simulink model "21-E"  (R2014a)
settings: Solver=FixedStepDiscrete  StartTime=0.0  StopTime=10.0  FixedStep=0.0005  RelTol=1e-3
undefined symbols (not defined in the file): add_k1_100, add_k2_100, ADDspeed, cal_acc_div, cal_acc_flo_add, cal_acc_min, cal_an_div, cal_an_min, cal_bre_div, cal_bre_en_add, cal_bre_flo_add, cal_bre_min, cal_conf_off, cal_conf_on, controller, ecucoder_acal, enres_on_add, enres_per_add
libraries: simulink x165, ec55xxlib x29
(part 3 of 6)

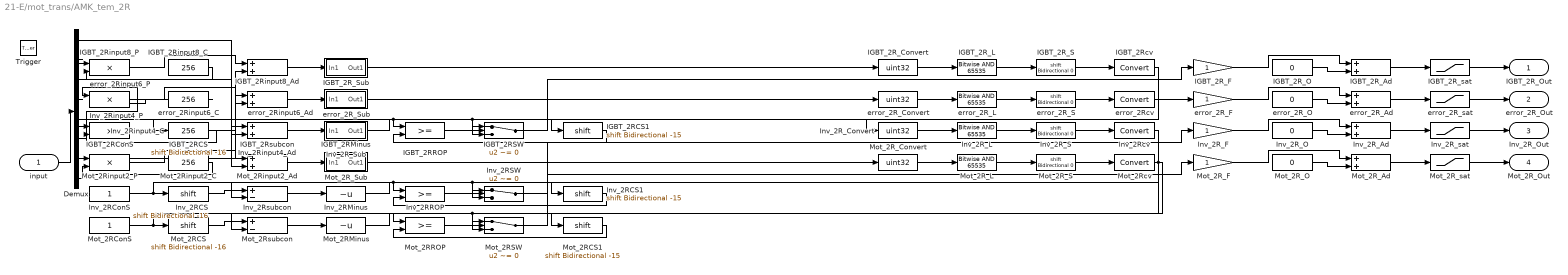
== system 21-E/mot_trans/AMK_tem_2R ==
  input : Inport
  Trigger : TriggerPort  TriggerType=function-call  PortDimensions=1
  Demux : Demux  Outputs=8
  IGBT_2RCS : ArithShift  BitShiftNumber=-16
  IGBT_2RCS1 : ArithShift  BitShiftNumber=-15
  IGBT_2RConS : Constant  OutDataTypeStr=single
  IGBT_2RMinus : UnaryMinus
  IGBT_2RROP : RelationalOperator  OutDataTypeStr=boolean
  IGBT_2RSW : Switch  Criteria=u2 ~= 0
  IGBT_2R_Ad : Sum
  IGBT_2R_Convert : DataTypeConversion  OutDataTypeStr=uint32
  IGBT_2R_F : Gain
  IGBT_2R_L : simulink/Logic and Bit Operations/Bitwise Operator  logicop=AND  UseBitMask=on  BitMask=65535  BitMaskRealWorld=Stored Integer
  IGBT_2R_O : Constant  Value=0  OutDataTypeStr=single
  IGBT_2R_S : ArithShift
  IGBT_2R_Sub : Subsystem
  IGBT_2R_sat : Saturate  UpperLimit=32767  LowerLimit=-32768
  IGBT_2Rcv : DataTypeConversion
  IGBT_2Rinput8_Ad : Sum
  IGBT_2Rinput8_C : Constant  Value=256
  IGBT_2Rinput8_P : Product
  IGBT_2Rsubcon : Sum  Inputs=+-
  Inv_2RCS : ArithShift  BitShiftNumber=-16
  Inv_2RCS1 : ArithShift  BitShiftNumber=-15
  Inv_2RConS : Constant  OutDataTypeStr=single
  Inv_2RMinus : UnaryMinus
  Inv_2RROP : RelationalOperator  OutDataTypeStr=boolean
  Inv_2RSW : Switch  Criteria=u2 ~= 0
  Inv_2R_Ad : Sum
  Inv_2R_Convert : DataTypeConversion  OutDataTypeStr=uint32
  Inv_2R_F : Gain
  Inv_2R_L : simulink/Logic and Bit Operations/Bitwise Operator  logicop=AND  UseBitMask=on  BitMask=65535  BitMaskRealWorld=Stored Integer
  Inv_2R_O : Constant  Value=0  OutDataTypeStr=single
  Inv_2R_S : ArithShift
  Inv_2R_Sub : Subsystem
  Inv_2R_sat : Saturate  UpperLimit=32767  LowerLimit=-32768
  Inv_2Rcv : DataTypeConversion
  Inv_2Rinput4_Ad : Sum
  Inv_2Rinput4_C : Constant  Value=256
  Inv_2Rinput4_P : Product
  Inv_2Rsubcon : Sum  Inputs=+-
  Mot_2RCS : ArithShift  BitShiftNumber=-16
  Mot_2RCS1 : ArithShift  BitShiftNumber=-15
  Mot_2RConS : Constant  OutDataTypeStr=single
  Mot_2RMinus : UnaryMinus
  Mot_2RROP : RelationalOperator  OutDataTypeStr=boolean
  Mot_2RSW : Switch  Criteria=u2 ~= 0
  Mot_2R_Ad : Sum
  Mot_2R_Convert : DataTypeConversion  OutDataTypeStr=uint32
  Mot_2R_F : Gain
  Mot_2R_L : simulink/Logic and Bit Operations/Bitwise Operator  logicop=AND  UseBitMask=on  BitMask=65535  BitMaskRealWorld=Stored Integer
  Mot_2R_O : Constant  Value=0  OutDataTypeStr=single
  Mot_2R_S : ArithShift
  Mot_2R_Sub : Subsystem
  Mot_2R_sat : Saturate  UpperLimit=32767  LowerLimit=-32768
  Mot_2Rcv : DataTypeConversion
  Mot_2Rinput2_Ad : Sum
  Mot_2Rinput2_C : Constant  Value=256
  Mot_2Rinput2_P : Product
  Mot_2Rsubcon : Sum  Inputs=+-
  error_2R_Ad : Sum
  error_2R_Convert : DataTypeConversion  OutDataTypeStr=uint32
  error_2R_F : Gain
  error_2R_L : simulink/Logic and Bit Operations/Bitwise Operator  logicop=AND  UseBitMask=on  BitMask=65535  BitMaskRealWorld=Stored Integer
  error_2R_O : Constant  Value=0  OutDataTypeStr=single
  error_2R_S : ArithShift
  error_2R_Sub : Subsystem
  error_2R_sat : Saturate  UpperLimit=65535  LowerLimit=0
  error_2Rcv : DataTypeConversion
  error_2Rinput6_Ad : Sum
  error_2Rinput6_C : Constant  Value=256
  error_2Rinput6_P : Product
  IGBT_2R_Out : Outport
  error_2R_Out : Outport  Port=2
  Inv_2R_Out : Outport  Port=3
  Mot_2R_Out : Outport  Port=4
  wires:
  input/1 -> Demux/1
  Mot_2RROP/1 -> Mot_2RSW/2
  Mot_2RSW/1 -> Mot_2R_F/1
  Mot_2RMinus/1 -> Mot_2RSW/1
  Mot_2Rsubcon/1 -> Mot_2RMinus/1
  Mot_2RCS/1 -> Mot_2Rsubcon/1
  Mot_2RCS1/1 -> Mot_2RROP/2
  Mot_2RConS/1 -> Mot_2RCS1/1, Mot_2RCS/1
  Mot_2Rcv/1 -> Mot_2RSW/3, Mot_2Rsubcon/2, Mot_2RROP/1
  Mot_2R_S/1 -> Mot_2Rcv/1
  Mot_2R_L/1 -> Mot_2R_S/1
  Mot_2R_Convert/1 -> Mot_2R_L/1
  Mot_2R_Sub/1(Out1) -> Mot_2R_Convert/1
  Mot_2Rinput2_Ad/1 -> Mot_2R_Sub/1(In1)
  Demux/1 -> Mot_2Rinput2_Ad/2
  Mot_2Rinput2_P/1 -> Mot_2Rinput2_Ad/1
  Mot_2Rinput2_C/1 -> Mot_2Rinput2_P/2
  Demux/2 -> Mot_2Rinput2_P/1
  Mot_2R_sat/1 -> Mot_2R_Out/1
  Mot_2R_Ad/1 -> Mot_2R_sat/1
  Mot_2R_O/1 -> Mot_2R_Ad/2
  Mot_2R_F/1 -> Mot_2R_Ad/1
  Inv_2RROP/1 -> Inv_2RSW/2
  Inv_2RSW/1 -> Inv_2R_F/1
  Inv_2RMinus/1 -> Inv_2RSW/1
  Inv_2Rsubcon/1 -> Inv_2RMinus/1
  Inv_2RCS/1 -> Inv_2Rsubcon/1
  Inv_2RCS1/1 -> Inv_2RROP/2
  Inv_2RConS/1 -> Inv_2RCS1/1, Inv_2RCS/1
  Inv_2Rcv/1 -> Inv_2Rsubcon/2, Inv_2RROP/1, Inv_2RSW/3
  Inv_2R_S/1 -> Inv_2Rcv/1
  Inv_2R_L/1 -> Inv_2R_S/1
  Inv_2R_Convert/1 -> Inv_2R_L/1
  Inv_2R_Sub/1(Out1) -> Inv_2R_Convert/1
  Inv_2Rinput4_Ad/1 -> Inv_2R_Sub/1(In1)
  Demux/3 -> Inv_2Rinput4_Ad/2
  Inv_2Rinput4_P/1 -> Inv_2Rinput4_Ad/1
  Inv_2Rinput4_C/1 -> Inv_2Rinput4_P/2
  Demux/4 -> Inv_2Rinput4_P/1
  Inv_2R_sat/1 -> Inv_2R_Out/1
  Inv_2R_Ad/1 -> Inv_2R_sat/1
  Inv_2R_O/1 -> Inv_2R_Ad/2
  Inv_2R_F/1 -> Inv_2R_Ad/1
  error_2Rcv/1 -> error_2R_F/1
  error_2R_S/1 -> error_2Rcv/1
  error_2R_L/1 -> error_2R_S/1
  error_2R_Convert/1 -> error_2R_L/1
  error_2R_Sub/1(Out1) -> error_2R_Convert/1
  error_2Rinput6_Ad/1 -> error_2R_Sub/1(In1)
  Demux/5 -> error_2Rinput6_Ad/2
  error_2Rinput6_P/1 -> error_2Rinput6_Ad/1
  error_2Rinput6_C/1 -> error_2Rinput6_P/2
  Demux/6 -> error_2Rinput6_P/1
  error_2R_sat/1 -> error_2R_Out/1
  error_2R_Ad/1 -> error_2R_sat/1
  error_2R_O/1 -> error_2R_Ad/2
  error_2R_F/1 -> error_2R_Ad/1
  IGBT_2RROP/1 -> IGBT_2RSW/2
  IGBT_2RSW/1 -> IGBT_2R_F/1
  IGBT_2RMinus/1 -> IGBT_2RSW/1
  IGBT_2Rsubcon/1 -> IGBT_2RMinus/1
  IGBT_2RCS/1 -> IGBT_2Rsubcon/1
  IGBT_2RCS1/1 -> IGBT_2RROP/2
  IGBT_2RConS/1 -> IGBT_2RCS1/1, IGBT_2RCS/1
  IGBT_2Rcv/1 -> IGBT_2Rsubcon/2, IGBT_2RROP/1, IGBT_2RSW/3
  IGBT_2R_S/1 -> IGBT_2Rcv/1
  IGBT_2R_L/1 -> IGBT_2R_S/1
  IGBT_2R_Convert/1 -> IGBT_2R_L/1
  IGBT_2R_Sub/1(Out1) -> IGBT_2R_Convert/1
  IGBT_2Rinput8_Ad/1 -> IGBT_2R_Sub/1(In1)
  Demux/7 -> IGBT_2Rinput8_Ad/2
  IGBT_2Rinput8_P/1 -> IGBT_2Rinput8_Ad/1
  IGBT_2Rinput8_C/1 -> IGBT_2Rinput8_P/2
  Demux/8 -> IGBT_2Rinput8_P/1
  IGBT_2R_sat/1 -> IGBT_2R_Out/1
  IGBT_2R_Ad/1 -> IGBT_2R_sat/1
  IGBT_2R_O/1 -> IGBT_2R_Ad/2
  IGBT_2R_F/1 -> IGBT_2R_Ad/1

== system 21-E/mot_trans/Subsystem ==
  ome : Inport
  Constant : Constant  Value=2*pi/60
  Constant5 : Constant  Value=0.225
  Gain : Gain  Gain=1/12.5
  Product : Product
  Product1 : Product
  v : Outport
  wires:
  ome/1 -> Product/1
  Product/1 -> Product1/1
  Constant5/1 -> Product1/2
  Product1/1 -> Gain/1
  Constant/1 -> Product/2
  Gain/1 -> v/1

== system 21-E/mot_trans/Subsystem1 ==
  ome : Inport
  Constant : Constant  Value=2*pi/60
  Constant5 : Constant  Value=0.225
  Gain : Gain  Gain=1/12.5
  Product : Product
  Product1 : Product
  v : Outport
  wires:
  Constant/1 -> Product/2
  Product1/1 -> Gain/1
  Constant5/1 -> Product1/2
  Product/1 -> Product1/1
  ome/1 -> Product/1
  Gain/1 -> v/1

== system 21-E/mot_trans/Subsystem2 ==
  ome : Inport
  Constant : Constant  Value=2*pi/60
  Constant5 : Constant  Value=0.225
  Gain : Gain  Gain=1/12.5
  Product : Product
  Product1 : Product
  v : Outport
  wires:
  Constant/1 -> Product/2
  Product1/1 -> Gain/1
  Constant5/1 -> Product1/2
  Product/1 -> Product1/1
  ome/1 -> Product/1
  Gain/1 -> v/1

== system 21-E/mot_trans/Subsystem4 ==
  ome : Inport
  Constant : Constant  Value=2*pi/60
  Constant5 : Constant  Value=0.225
  Gain : Gain  Gain=1/12.5
  Product : Product
  Product1 : Product
  v : Outport
  wires:
  Gain/1 -> v/1
  ome/1 -> Product/1
  Product/1 -> Product1/1
  Constant5/1 -> Product1/2
  Product1/1 -> Gain/1
  Constant/1 -> Product/2

== system 21-E/run/Subsystem ==
  note: 输出给各个轮胎的绝对值负转矩Nm
  note: 电机应提供的总制动力距
  note: 理想的前后轴分配比
  note: 前轮卡钳制动力
  note: 目标制动力矩
  note: 目标减速度
  note: 开度
  note: 注：压力变送器最大误差0.075Mpa
  note: 后轮卡钳制动力
  bra signal : Inport
  "pressure sensor_front（pa） " : Inport  Port=2
  "pressure sensor_rear（pa） " : Inport  Port=3
  Constant : Constant
  Data Type Conversion : DataTypeConversion  OutDataTypeStr=double
  Data Type Conversion1 : DataTypeConversion  OutDataTypeStr=double
  Fcn1 : Fcn  Expr=u(1)*u(2)
  Fcn2 : Fcn  Expr=(u(2)-u(1))*u(3)
  Gain : Gain  Gain=0.5
  Gain1 : Gain  Gain=0.5
  Gain2 : Gain  Gain=0.5
  M1 : Constant  Value=310
  Mux{,1..2,4..5} (5 alike) : Mux  Inputs=2
  Mux3 : Mux  Inputs=3
  Mux6 : Mux  Inputs=3
  Switch : Switch  Criteria=u2 > Threshold  Threshold=500000
  Switch1 : Switch  Criteria=u2 > Threshold  Threshold=500000
  Torque_bf : Fcn  Expr=u(1)*u(2)*0.35*0.025*0.025
  Torque_br : Fcn  Expr=u(1)*u(2)*0.025*0.025*0.35*0.5
  aim acceleration : MATLAB Function  TreatAsAtomicUnit=on
  aim brake Torque : Fcn  Expr=u(1)*u(2)*9.8/0.225
  "brake disc_Re(m) " : Constant  Value=0.097
  "mechanica ratio " : Fcn  Expr=u(1)/(u(1)+u(2))
  "total motor Torque " : Fcn  Expr=u(3)-u(2)-u(1)
  "FL motor Torque " : Outport
  FR motor Torque : Outport  Port=2
  RL motor Torque : Outport  Port=3
  RR motor Torque1 : Outport  Port=4
  wires:
  Mux/1 -> Torque_bf/1
  "pressure sensor_front（pa） "/1 -> Mux/1
  "brake disc_Re(m) "/1 -> Mux1/1, Mux/2
  bra signal/1 -> aim acceleration/1(x)
  Mux4/1 -> "mechanica ratio "/1
  Gain1/1 -> FR motor Torque/1, "FL motor Torque "/1
  "mechanica ratio "/1 -> Data Type Conversion/1
  Mux5/1 -> Fcn1/1
  Mux2/1 -> aim brake Torque/1
  aim acceleration/1(g) -> Mux2/1
  aim brake Torque/1 -> Mux3/3
  Data Type Conversion1/1 -> Mux5/1, Mux6/3, Gain/1
  Fcn1/1 -> Switch/1
  Constant/1 -> Mux6/2
  Gain/1 -> Switch1/3, Switch/3
  Fcn2/1 -> Switch1/1
  Gain2/1 -> RR motor Torque1/1, RL motor Torque/1
  M1/1 -> Mux2/2
  Torque_br/1 -> Mux4/2, Mux3/2
  Torque_bf/1 -> Mux3/1, Mux4/1
  "pressure sensor_rear（pa） "/1 -> Switch1/2, Switch/2, Mux1/2
  Mux6/1 -> Fcn2/1
  "total motor Torque "/1 -> Data Type Conversion1/1
  Switch/1 -> Gain1/1
  Data Type Conversion/1 -> Mux6/1, Mux5/2
  Mux1/1 -> Torque_br/1
  Switch1/1 -> Gain2/1
  Mux3/1 -> "total motor Torque "/1

== system 21-E/run/analog_acq ==
  AnalogInput : ec55xxlib/RapidECU_U1/02AnalogInput/AnalogInput  channel=75: I_AN21_5V  sampletime=-1
  AnalogInput1 : ec55xxlib/RapidECU_U1/02AnalogInput/AnalogInput  channel=73: I_AN19_5V  sampletime=-1
  AnalogInput2 : ec55xxlib/RapidECU_U1/02AnalogInput/AnalogInput  channel=54: I_AN15_5V  sampletime=-1
  AnalogInput3 : ec55xxlib/RapidECU_U1/02AnalogInput/AnalogInput  channel=55: I_AN16_5V  sampletime=-1
  Constant : Constant  Value=5000
  Constant1 : Constant  Value=15
  Constant2 : Constant  Value=5000
  Constant3 : Constant  Value=15
  Data Store Read : DataStoreRead  DataStoreName=sensor_acc
  Data Store Read1 : DataStoreRead  DialogController=Simulink.DDGSource  DataStoreName=sensor_bre
  Data Store Read2 : DataStoreRead  Priority=0  DialogController=Simulink.DDGSource  DataStoreName=enable
  Data Store Write1 : DataStoreWrite  Priority=0  DataStoreName=sensor_acc
  Data Store Write2 : DataStoreWrite  Priority=0  DataStoreName=sensor_bre
  Data Store Write3 : DataStoreWrite  Priority=1  DialogController=Simulink.DDGSource  DataStoreName=enable
  Data Store Write4 : DataStoreWrite  Priority=0  DialogController=Simulink.DDGSource  DataStoreName=oil1
  Data Store Write5 : DataStoreWrite  Priority=0  DataStoreName=oil2
  Data Type Conversion : DataTypeConversion  OutDataTypeStr=boolean
  Data Type Conversion1 : DataTypeConversion  OutDataTypeStr=boolean
  Data Type Conversion2 : DataTypeConversion  OutDataTypeStr=boolean
  Gain : Gain  Gain=1e6
  Gain1 : Gain  Gain=1e6
  Logical Operator : Logic  Operator=NOT  AllPortsSameDT=off  OutDataTypeStr=boolean
  Logical Operator1 : Logic  Operator=NOT  AllPortsSameDT=off  OutDataTypeStr=boolean
  MATLAB Function : MATLAB Function  TreatAsAtomicUnit=on
  MATLAB Function1 : MATLAB Function  TreatAsAtomicUnit=on
  MATLAB Function2 : MATLAB Function  TreatAsAtomicUnit=on
  Product : Product  Inputs=*/*
  Product1 : Product  Inputs=*/*
  jud_acc : Subsystem
  jud_bre : Subsystem
  acc_ana : Outport
  bre_ana : Outport  Port=2
  oilpre1 : Outport  Port=3
  oilpre2 : Outport  Port=4
  wires:
  AnalogInput/1 -> bre_ana/1, jud_bre/1(In1)  "ori_bre_li"
  AnalogInput1/1 -> acc_ana/1, jud_acc/1(In1)  "ori_acc_li"
  jud_acc/1(Out1) -> MATLAB Function1/1(u)
  Logical Operator/1 -> Data Type Conversion/1  "sensor_acc"
  Logical Operator1/1 -> Data Type Conversion1/1  "sensor_bre"
  jud_bre/1(Out1) -> MATLAB Function2/1(u)
  Data Store Read/1 -> MATLAB Function/1(x)
  Data Store Read1/1 -> MATLAB Function/2(y)
  Data Store Read2/1 -> MATLAB Function/3(d_)
  MATLAB Function/1(d) -> Data Type Conversion2/1
  MATLAB Function1/1(y) -> Logical Operator/1
  MATLAB Function2/1(y) -> Logical Operator1/1
  Data Type Conversion/1 -> Data Store Write1/1
  Data Type Conversion1/1 -> Data Store Write2/1
  Data Type Conversion2/1 -> Data Store Write3/1
  AnalogInput2/1 -> Product/1  "oil_pre_1"
  AnalogInput3/1 -> Product1/1  "oil_pre_2"
  Constant/1 -> Product/2
  Constant1/1 -> Product/3
  Constant2/1 -> Product1/2
  Constant3/1 -> Product1/3
  Product/1 -> Gain/1
  Gain/1 -> Data Store Write4/1, oilpre1/1
  Product1/1 -> Gain1/1
  Gain1/1 -> Data Store Write5/1, oilpre2/1

== system 21-E/run/cal&con ==
  acc_ana : Inport
  bre_ana : Inport  Port=2
  Add : Sum  Inputs=+-
  Add{1..3,5..6,8..9} (7 alike) : Sum  Inputs=2
  Add4 : Sum  Inputs=+-
  Add7 : Sum  Inputs=-+
  Constant : Constant  Value=0.25
  Constant1 : Constant  Value=0.3
  Constant11 : Constant  Value=400000
  Constant12 : Constant  Value=400000  OutDataTypeStr=uint32
  Constant2 : Constant  Value=0.15
  Constant3 : Constant  Value=0.2
  Constant4 : Constant
  Constant5 : Constant  Value=2650
  Constant6 : Constant  Value=1650
  Constant7 : Constant  Value=0.3
  Constant8 : Constant  Value=350
  Constant9 : Constant  Value=2100
  Data Store Write2 : DataStoreWrite  Priority=0  DialogController=Simulink.DDGSource  DataStoreName=enable_bre
  Data Type Conversion1 : DataTypeConversion  OutDataTypeStr=uint32
  Divide : Product  Inputs=*/
  Divide1 : Product  Inputs=*/
  Divide2 : Product
  ECCalVar : Constant  InitFcn=ecucoder_acal;  Value=cal_bre_min  OutDataTypeStr=Inherit: Inherit via back propagation  SampleTime=-1
  ECCalVar1 : Constant  InitFcn=ecucoder_acal;  Value=cal_bre_en_add  OutDataTypeStr=Inherit: Inherit via back propagation  SampleTime=-1
  ECCalVar2 : Constant  InitFcn=ecucoder_acal;  Value=cal_bre_div  OutDataTypeStr=Inherit: Inherit via back propagation  SampleTime=-1
  ECCalVar3 : Constant  InitFcn=ecucoder_acal;  Value=cal_acc_min  OutDataTypeStr=Inherit: Inherit via back propagation  SampleTime=-1
  ECCalVar4 : Constant  InitFcn=ecucoder_acal;  Value=cal_conf_on  OutDataTypeStr=Inherit: Inherit via back propagation  SampleTime=-1
  ECCalVar5 : Constant  InitFcn=ecucoder_acal;  Value=cal_acc_div  OutDataTypeStr=Inherit: Inherit via back propagation  SampleTime=-1
  ECCalVar6 : Constant  InitFcn=ecucoder_acal;  Value=cal_conf_off  OutDataTypeStr=Inherit: Inherit via back propagation  SampleTime=-1
  Logical Operator : Logic  AllPortsSameDT=off  OutDataTypeStr=boolean
  Logical Operator3 : Logic  AllPortsSameDT=off  OutDataTypeStr=boolean
  MATLAB Function2 : MATLAB Function  TreatAsAtomicUnit=on
  PowerDriverPWM : ec55xxlib/RapidECU_U1/06PowerDriverPWM/PowerDriverPWM  channel=115: O_PWM10_HS2A9  sampletime=-1
  Relational Operator : RelationalOperator  OutDataTypeStr=boolean
  Relational Operator1 : RelationalOperator  OutDataTypeStr=boolean
  Relational Operator2 : RelationalOperator  Operator=<=  OutDataTypeStr=boolean
  Relational Operator3 : RelationalOperator  OutDataTypeStr=boolean
  Relational Operator4 : RelationalOperator  Operator=<=  OutDataTypeStr=boolean
  Saturation : Saturate  UpperLimit=5000  LowerLimit=0
  Saturation1 : Saturate  UpperLimit=5000  LowerLimit=0
  Saturation2 : Saturate  UpperLimit=1  LowerLimit=0
  Saturation3 : Saturate  UpperLimit=1  LowerLimit=0
  can_conf : Subsystem
  conf : Subsystem
  acc : Outport
  bre : Outport  Port=2
  wires:
  Add4/1 -> Divide1/1  "calacc_min"
  ECCalVar5/1 -> Add6/2
  Add6/1 -> Divide1/2  "calacc_div"
  Constant9/1 -> Add6/1
  Add5/1 -> Add4/2
  Constant8/1 -> Add5/1
  ECCalVar3/1 -> Add5/2
  Divide1/1 -> Saturation2/1  "acc_cal"
  Saturation/1 -> Add4/1
  Add/1 -> Divide/1  "calbre_min"
  Divide/1 -> Saturation3/1  "bre_cal"
  Relational Operator3/1 -> Data Store Write2/1  "en_bre"
  ECCalVar2/1 -> Add2/2
  Add2/1 -> Divide/2  "calbre_div"
  Constant6/1 -> Add2/1
  Add1/1 -> Add/2
  Constant5/1 -> Add1/1
  ECCalVar/1 -> Add1/2
  Constant7/1 -> Add3/1
  ECCalVar1/1 -> Add3/2
  Saturation1/1 -> Add/1
  Logical Operator/1 -> conf/Enable
  Relational Operator1/1 -> Logical Operator/2
  Constant2/1 -> Relational Operator2/2
  Relational Operator/1 -> Logical Operator/1
  Relational Operator2/1 -> Logical Operator3/1
  Constant/1 -> Relational Operator/2
  Saturation2/1 -> Relational Operator2/1, Relational Operator/1, acc/1  "acc_sat"
  Logical Operator3/1 -> can_conf/Enable
  Relational Operator4/1 -> Logical Operator3/2
  Saturation3/1 -> Add7/1
  Constant4/1 -> Add7/2
  Add7/1 -> MATLAB Function2/1(bre), Relational Operator3/1, Relational Operator4/1, Relational Operator1/1, bre/1  "bre_sat"
  Add3/1 -> Relational Operator3/2
  acc_ana/1 -> Saturation/1
  bre_ana/1 -> Saturation1/1
  Constant1/1 -> Add8/1
  Add8/1 -> Relational Operator1/2  "calconf_on"
  ECCalVar4/1 -> Add8/2
  Add9/1 -> Relational Operator4/2  "calconf_off"
  ECCalVar6/1 -> Add9/2
  Constant3/1 -> Add9/1
  Divide2/1 -> Data Type Conversion1/1
  Constant12/1 -> PowerDriverPWM/1
  MATLAB Function2/1(tri_lig) -> Divide2/1  "tri_lig"
  Data Type Conversion1/1 -> PowerDriverPWM/2
  Constant11/1 -> Divide2/2

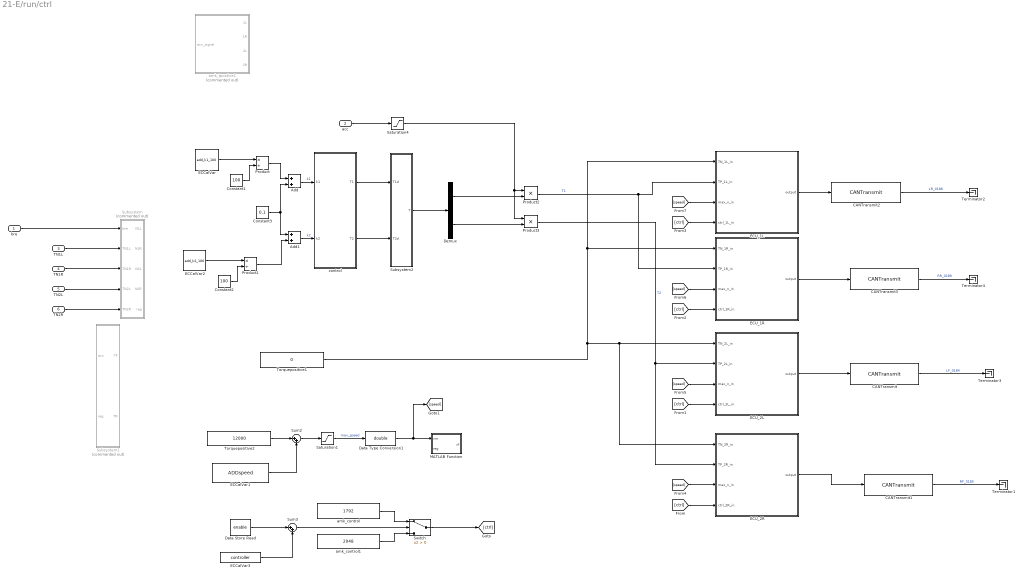
== system 21-E/run/ctrl ==
  bre : Inport
  acc : Inport  Port=2
  TN1L : Inport  Port=3
  TN1R : Inport  Port=4
  TN2L : Inport  Port=5
  TN2R : Inport  Port=6
  Add : Sum
  Add1 : Sum
  CANTransmit : ec55xxlib/RapidECU_U2/07CANCommucation/CANTransmit  canmodule=A  canbuffer=9  canmessageid=hex2dec('0184')  canmessagetype=Standard(11-bit ID)  datalength=8  sampletime=-1
  CANTransmit1 : ec55xxlib/RapidECU_U2/07CANCommucation/CANTransmit  canmodule=A  canbuffer=10  canmessageid=hex2dec('0185')  canmessagetype=Standard(11-bit ID)  datalength=8  sampletime=-1
  CANTransmit2 : ec55xxlib/RapidECU_U2/07CANCommucation/CANTransmit  canmodule=A  canbuffer=11  canmessageid=hex2dec('0188')  canmessagetype=Standard(11-bit ID)  datalength=8  sampletime=-1
  CANTransmit3 : ec55xxlib/RapidECU_U2/07CANCommucation/CANTransmit  canmodule=A  canbuffer=12  canmessageid=hex2dec('0189')  canmessagetype=Standard(11-bit ID)  datalength=8  sampletime=-1
  Constant1 : Constant  Value=100
  Constant2 : Constant  Value=100
  Constant3 : Constant  Value=0.1
  Data Store Read : DataStoreRead  DialogController=Simulink.DDGSource  DataStoreName=enable
  Data Type Conversion1 : DataTypeConversion  OutDataTypeStr=double
  Demux : Demux  Outputs=2
  ECCalVar : Constant  InitFcn=ecucoder_acal;  Value=add_k1_100  OutDataTypeStr=Inherit: Inherit via back propagation  SampleTime=-1
  ECCalVar1 : Constant  InitFcn=ecucoder_acal;  Value=ADDspeed  OutDataTypeStr=Inherit: Inherit via back propagation  SampleTime=-1
  ECCalVar2 : Constant  InitFcn=ecucoder_acal;  Value=add_k2_100  OutDataTypeStr=Inherit: Inherit via back propagation  SampleTime=-1
  ECCalVar3 : Constant  InitFcn=ecucoder_acal;  Value=controller  OutDataTypeStr=Inherit: Inherit via back propagation  SampleTime=-1
  ECU_1L : Subsystem
  ECU_1R : Subsystem
  ECU_2L : Subsystem
  ECU_2R : Subsystem
  MATLAB Function : MATLAB Function  TreatAsAtomicUnit=on
  Product : Product  Inputs=*/
  Product1 : Product  Inputs=*/
  Product2 : Product
  Product3 : Product
  Saturation1 : Saturate  UpperLimit=15000  LowerLimit=0
  Saturation4 : Saturate  UpperLimit=1  LowerLimit=0
  Subsystem : Subsystem  Commented=on
  Subsystem1 : Subsystem  Commented=on
  Subsystem2 : Subsystem
  Sum2 : Sum  Inputs=|++
  Sum3 : Sum  Inputs=|++
  Switch : Switch  Criteria=u2 > Threshold
  Terminator{1..4} (4 alike) : Terminator
  Torquepositive1 : Constant  Value=0
  Torquepositive2 : Constant  Value=12000
  amk_control : Constant  Value=1792
  amk_control1 : Constant  Value=2048
  amk_tpostive1 : Subsystem  Commented=on
  control : Subsystem
  wires:
  Sum2/1 -> Saturation1/1
  Torquepositive2/1 -> Sum2/1
  ECCalVar1/1 -> Sum2/2
  Saturation1/1 -> Data Type Conversion1/1  "max_speed"
  Data Store Read/1 -> Sum3/1
  ECCalVar3/1 -> Sum3/2
  amk_control/1 -> Switch/1
  amk_control1/1 -> Switch/3
  CANTransmit1/1 -> Terminator1/1  "RF_0185"
  CANTransmit/1 -> Terminator3/1  "LF_0184"
  CANTransmit2/1 -> Terminator2/1  "LR_0188"
  CANTransmit3/1 -> Terminator4/1  "RR_0189"
  Sum3/1 -> Switch/2
  Switch/1 -> [ctrl]
  [ctrl] -> ECU_2R/4(ctrl_2R_in)
  [ctrl] -> ECU_2L/4(ctrl_2L_in)
  [ctrl] -> ECU_1R/4(ctrl_1R_in)
  [ctrl] -> ECU_1L/4(ctrl_1L_in)
  [speed] -> ECU_2R/3(max_n_in)
  [speed] -> ECU_2L/3(max_n_in)
  [speed] -> ECU_1R/3(max_n_in)
  [speed] -> ECU_1L/3(max_n_in)
  bre/1 -> Subsystem/1(bre)
  TN1L/1 -> Subsystem/2(TN1L)
  TN2L/1 -> Subsystem/4(TN2L)
  TN2R/1 -> Subsystem/5(TN2R)
  TN1R/1 -> Subsystem/3(TN1R)
  Data Type Conversion1/1 -> [speed], MATLAB Function/1(vm)
  Torquepositive1/1 -> ECU_1L/1(TN_1L_in), ECU_1R/1(TN_1R_in), ECU_2R/1(TN_2R_in), ECU_2L/1(TN_2L_in)
  ECU_1L/1(output) -> CANTransmit2/1
  ECU_1R/1(output) -> CANTransmit3/1
  ECU_2L/1(output) -> CANTransmit/1
  ECU_2R/1(output) -> CANTransmit1/1
  Add/1 -> control/1(k1)  "k1"
  ECCalVar/1 -> Product/1
  Product/1 -> Add/1
  Constant1/1 -> Product/2
  ECCalVar2/1 -> Product1/1
  Product1/1 -> Add1/2
  Constant2/1 -> Product1/2
  Add1/1 -> control/2(k2)  "k2"
  Constant3/1 -> Add1/1, Add/2
  Saturation4/1 -> Product3/1, Product2/1
  control/1(T1) -> Subsystem2/1(T1d)
  control/2(T2) -> Subsystem2/2(T2d)
  Subsystem2/1(T) -> Demux/1
  Demux/1 -> Product2/2
  Demux/2 -> Product3/2
  acc/1 -> Saturation4/1
  Product2/1 -> ECU_1R/2(TP_1R_in), ECU_1L/2(TP_1L_in)  "T1"
  Product3/1 -> ECU_2R/2(TP_2R_in), ECU_2L/2(TP_2L_in)  "T2"

== system 21-E/run/emp ==
  acc : Inport
  bre : Inport  Port=2
  Add : Sum  Inputs=+-
  Add1 : Sum  Inputs=+-
  Constant3 : Constant  Value=0  OutDataTypeStr=double
  Constant4 : Constant  OutDataTypeStr=double
  Constant5 : Constant  Value=0.1  OutDataTypeStr=double
  Constant6 : Constant  Value=0.9  OutDataTypeStr=double
  Constant8 : Constant  Value=0.8  OutDataTypeStr=double
  Constant9 : Constant  Value=0.1  OutDataTypeStr=double
  Data Store Read : DataStoreRead  DialogController=Simulink.DDGSource  DataStoreName=enable
  Data Store Read1 : DataStoreRead  DataStoreName=pedal_con
  Data Store Read2 : DataStoreRead  DialogController=Simulink.DDGSource  DataStoreName=sensor_acc
  Data Store Read3 : DataStoreRead  DialogController=Simulink.DDGSource  DataStoreName=sensor_bre
  Data Store Write : DataStoreWrite  DataStoreName=acc_signal
  Data Store Write1 : DataStoreWrite  DialogController=Simulink.DDGSource  DataStoreName=break_signal
  Divide : Product  Inputs=*/
  Divide1 : Product  Inputs=*/
  Logical Operator1 : Logic  Operator=NOT  AllPortsSameDT=off  OutDataTypeStr=boolean
  Logical Operator2 : Logic  Inputs=4  AllPortsSameDT=off  OutDataTypeStr=boolean
  Saturation : Saturate  UpperLimit=0.9  LowerLimit=0
  Saturation1 : Saturate  UpperLimit=1  LowerLimit=0
  Saturation2 : Saturate  UpperLimit=0.8  LowerLimit=0
  Saturation3 : Saturate  UpperLimit=1  LowerLimit=0
  bre_fin : Outport
  acc_fin : Outport  Port=2
  wires:
  Data Store Read/1 -> Logical Operator2/1
  Data Store Read1/1 -> Logical Operator1/1  "ped_con"
  Logical Operator1/1 -> Logical Operator2/2
  Data Store Read2/1 -> Logical Operator2/3
  Data Store Read3/1 -> Logical Operator2/4
  Divide1/1 -> Saturation3/1  "bre_emp"
  Saturation1/1 -> acc_fin/1, Data Store Write/1  "acc_emp"
  Add/1 -> Saturation/1
  Constant5/1 -> Add/2
  Saturation/1 -> Divide1/1
  Constant9/1 -> Add1/2
  Divide/1 -> Saturation1/1
  Constant6/1 -> Divide1/2
  Add1/1 -> Saturation2/1
  Saturation2/1 -> Divide/1
  Constant8/1 -> Divide/2
  acc/1 -> Add1/1
  bre/1 -> Add/1
  Saturation3/1 -> Data Store Write1/1, bre_fin/1

== system 21-E/waiting/Subsystem ==
  wait : Inport
  Add : Sum
  Add1 : Sum
  Constant2 : Constant  Value=600000  OutDataTypeStr=uint32
  Constant3 : Constant  Value=0  OutDataTypeStr=uint32
  Constant4 : Constant  Value=450000  OutDataTypeStr=uint32
  Constant5 : Constant  Value=0  OutDataTypeStr=uint32
  ECCalVar : Constant  InitFcn=ecucoder_acal;  Value=enres_per_add  OutDataTypeStr=uint32  SampleTime=-1
  ECCalVar1 : Constant  InitFcn=ecucoder_acal;  Value=enres_on_add  OutDataTypeStr=uint32  SampleTime=-1
  Switch : Switch  Criteria=u2 > Threshold
  Switch1 : Switch  Criteria=u2 > Threshold
  blow : ec55xxlib/RapidECU_U1/06PowerDriverPWM/PowerDriverPWM  channel=114: O_PWM9_HS2A9  sampletime=-1
  wires:
  Add1/1 -> Switch1/1
  Switch1/1 -> blow/2
  Switch/1 -> blow/1
  Constant4/1 -> Add1/2
  Constant5/1 -> Switch1/3
  Add/1 -> Switch/1
  Constant3/1 -> Switch/3
  Constant2/1 -> Add/2
  ECCalVar1/1 -> Add1/1
  ECCalVar/1 -> Add/1
  wait/1 -> Switch/2, Switch1/2

== system 21-E/waiting1/Subsystem ==
  wait : Inport
  Add : Sum
  Add1 : Sum
  Constant2 : Constant  Value=600000  OutDataTypeStr=uint32
  Constant3 : Constant  Value=0  OutDataTypeStr=uint32
  Constant4 : Constant  Value=450000  OutDataTypeStr=uint32
  Constant5 : Constant  Value=0  OutDataTypeStr=uint32
  ECCalVar : Constant  InitFcn=ecucoder_acal;  Value=enres_per_add  OutDataTypeStr=uint32  SampleTime=-1
  ECCalVar1 : Constant  InitFcn=ecucoder_acal;  Value=enres_on_add  OutDataTypeStr=uint32  SampleTime=-1
  Switch : Switch  Criteria=u2 > Threshold
  Switch1 : Switch  Criteria=u2 > Threshold
  blow : ec55xxlib/RapidECU_U1/06PowerDriverPWM/PowerDriverPWM  channel=114: O_PWM9_HS2A9  sampletime=-1
  wires:
  wait/1 -> Switch1/2, Switch/2
  ECCalVar/1 -> Add/1
  ECCalVar1/1 -> Add1/1
  Constant2/1 -> Add/2
  Constant3/1 -> Switch/3
  Add/1 -> Switch/1
  Constant5/1 -> Switch1/3
  Constant4/1 -> Add1/2
  Switch/1 -> blow/1
  Switch1/1 -> blow/2
  Add1/1 -> Switch1/1

== system 21-E/ECU_can/ECU_dyn1/s_1L ==
  s_1L : Inport
  Constant{1..3,5..8} (7 alike) : Constant  Value=0  OutDataTypeStr=uint8  SampleTime=-1
  s_1LRon : Rounding  Operator=round
  s_1L_1sat : Saturate  UpperLimit=255  LowerLimit=0
  s_1L_Convert : DataTypeConversion  OutDataTypeStr=uint8
  s_1L_Convert1 : DataTypeConversion  OutDataTypeStr=uint32
  s_1L_D : Product  Inputs=*/
  s_1L_F : Constant  OutDataTypeStr=single
  s_1L_L : simulink/Logic and Bit Operations/Bitwise Operator  logicop=AND  UseBitMask=on  BitMask=255  BitMaskRealWorld=Stored Integer
  s_1L_O : Constant  Value=0  OutDataTypeStr=single
  s_1L_S : ArithShift
  s_1L_sat : Saturate  UpperLimit=255  LowerLimit=0
  s_1L_st : Sum  Inputs=+-
  output1 : Outport
  output2 : Outport  Port=2
  output3 : Outport  Port=3
  output4 : Outport  Port=4
  output5 : Outport  Port=5
  output6 : Outport  Port=6
  output7 : Outport  Port=7
  output8 : Outport  Port=8
  wires:
  Constant8/1 -> output8/1
  Constant7/1 -> output7/1
  Constant6/1 -> output6/1
  Constant5/1 -> output5/1
  Constant3/1 -> output3/1
  Constant2/1 -> output2/1
  Constant1/1 -> output1/1
  s_1L_Convert/1 -> output4/1
  s_1L_L/1 -> s_1L_Convert/1
  s_1L_Convert1/1 -> s_1L_L/1
  s_1L_1sat/1 -> s_1L_Convert1/1
  s_1L_S/1 -> s_1L_1sat/1
  s_1LRon/1 -> s_1L_S/1
  s_1L_D/1 -> s_1LRon/1
  s_1L_F/1 -> s_1L_D/2
  s_1L_st/1 -> s_1L_D/1
  s_1L_O/1 -> s_1L_st/2
  s_1L_sat/1 -> s_1L_st/1
  s_1L/1 -> s_1L_sat/1

== system 21-E/ECU_can/ECU_dyn1/s_1R ==
  s_1R : Inport
  Constant{1..4,6..8} (7 alike) : Constant  Value=0  OutDataTypeStr=uint8  SampleTime=-1
  s_1RRon : Rounding  Operator=round
  s_1R_1sat : Saturate  UpperLimit=255  LowerLimit=0
  s_1R_Convert : DataTypeConversion  OutDataTypeStr=uint8
  s_1R_Convert1 : DataTypeConversion  OutDataTypeStr=uint32
  s_1R_D : Product  Inputs=*/
  s_1R_F : Constant  OutDataTypeStr=single
  s_1R_L : simulink/Logic and Bit Operations/Bitwise Operator  logicop=AND  UseBitMask=on  BitMask=255  BitMaskRealWorld=Stored Integer
  s_1R_O : Constant  Value=0  OutDataTypeStr=single
  s_1R_S : ArithShift
  s_1R_sat : Saturate  UpperLimit=255  LowerLimit=0
  s_1R_st : Sum  Inputs=+-
  output1 : Outport
  output2 : Outport  Port=2
  output3 : Outport  Port=3
  output4 : Outport  Port=4
  output5 : Outport  Port=5
  output6 : Outport  Port=6
  output7 : Outport  Port=7
  output8 : Outport  Port=8
  wires:
  Constant8/1 -> output8/1
  Constant7/1 -> output7/1
  Constant6/1 -> output6/1
  Constant4/1 -> output4/1
  Constant3/1 -> output3/1
  Constant2/1 -> output2/1
  Constant1/1 -> output1/1
  s_1R_Convert/1 -> output5/1
  s_1R_L/1 -> s_1R_Convert/1
  s_1R_Convert1/1 -> s_1R_L/1
  s_1R_1sat/1 -> s_1R_Convert1/1
  s_1R_S/1 -> s_1R_1sat/1
  s_1RRon/1 -> s_1R_S/1
  s_1R_D/1 -> s_1RRon/1
  s_1R_F/1 -> s_1R_D/2
  s_1R_st/1 -> s_1R_D/1
  s_1R_O/1 -> s_1R_st/2
  s_1R_sat/1 -> s_1R_st/1
  s_1R/1 -> s_1R_sat/1

== system 21-E/ECU_can/ECU_dyn1/s_2L ==
  s_2L : Inport
  Constant{1..5,7..8} (7 alike) : Constant  Value=0  OutDataTypeStr=uint8  SampleTime=-1
  s_2LRon : Rounding  Operator=round
  s_2L_1sat : Saturate  UpperLimit=255  LowerLimit=0
  s_2L_Convert : DataTypeConversion  OutDataTypeStr=uint8
  s_2L_Convert1 : DataTypeConversion  OutDataTypeStr=uint32
  s_2L_D : Product  Inputs=*/
  s_2L_F : Constant  OutDataTypeStr=single
  s_2L_L : simulink/Logic and Bit Operations/Bitwise Operator  logicop=AND  UseBitMask=on  BitMask=255  BitMaskRealWorld=Stored Integer
  s_2L_O : Constant  Value=0  OutDataTypeStr=single
  s_2L_S : ArithShift
  s_2L_sat : Saturate  UpperLimit=255  LowerLimit=0
  s_2L_st : Sum  Inputs=+-
  output1 : Outport
  output2 : Outport  Port=2
  output3 : Outport  Port=3
  output4 : Outport  Port=4
  output5 : Outport  Port=5
  output6 : Outport  Port=6
  output7 : Outport  Port=7
  output8 : Outport  Port=8
  wires:
  Constant8/1 -> output8/1
  Constant7/1 -> output7/1
  Constant5/1 -> output5/1
  Constant4/1 -> output4/1
  Constant3/1 -> output3/1
  Constant2/1 -> output2/1
  Constant1/1 -> output1/1
  s_2L_Convert/1 -> output6/1
  s_2L_L/1 -> s_2L_Convert/1
  s_2L_Convert1/1 -> s_2L_L/1
  s_2L_1sat/1 -> s_2L_Convert1/1
  s_2L_S/1 -> s_2L_1sat/1
  s_2LRon/1 -> s_2L_S/1
  s_2L_D/1 -> s_2LRon/1
  s_2L_F/1 -> s_2L_D/2
  s_2L_st/1 -> s_2L_D/1
  s_2L_O/1 -> s_2L_st/2
  s_2L_sat/1 -> s_2L_st/1
  s_2L/1 -> s_2L_sat/1

== system 21-E/ECU_can/ECU_dyn1/s_2R ==
  s_2R : Inport
  Constant{1..6,8} (7 alike) : Constant  Value=0  OutDataTypeStr=uint8  SampleTime=-1
  s_2RRon : Rounding  Operator=round
  s_2R_1sat : Saturate  UpperLimit=255  LowerLimit=0
  s_2R_Convert : DataTypeConversion  OutDataTypeStr=uint8
  s_2R_Convert1 : DataTypeConversion  OutDataTypeStr=uint32
  s_2R_D : Product  Inputs=*/
  s_2R_F : Constant  OutDataTypeStr=single
  s_2R_L : simulink/Logic and Bit Operations/Bitwise Operator  logicop=AND  UseBitMask=on  BitMask=255  BitMaskRealWorld=Stored Integer
  s_2R_O : Constant  Value=0  OutDataTypeStr=single
  s_2R_S : ArithShift
  s_2R_sat : Saturate  UpperLimit=255  LowerLimit=0
  s_2R_st : Sum  Inputs=+-
  output1 : Outport
  output2 : Outport  Port=2
  output3 : Outport  Port=3
  output4 : Outport  Port=4
  output5 : Outport  Port=5
  output6 : Outport  Port=6
  output7 : Outport  Port=7
  output8 : Outport  Port=8
  wires:
  Constant8/1 -> output8/1
  Constant6/1 -> output6/1
  Constant5/1 -> output5/1
  Constant4/1 -> output4/1
  Constant3/1 -> output3/1
  Constant2/1 -> output2/1
  Constant1/1 -> output1/1
  s_2R_Convert/1 -> output7/1
  s_2R_L/1 -> s_2R_Convert/1
  s_2R_Convert1/1 -> s_2R_L/1
  s_2R_1sat/1 -> s_2R_Convert1/1
  s_2R_S/1 -> s_2R_1sat/1
  s_2RRon/1 -> s_2R_S/1
  s_2R_D/1 -> s_2RRon/1
  s_2R_F/1 -> s_2R_D/2
  s_2R_st/1 -> s_2R_D/1
  s_2R_O/1 -> s_2R_st/2
  s_2R_sat/1 -> s_2R_st/1
  s_2R/1 -> s_2R_sat/1

== system 21-E/ECU_can/ECU_dyn1/slip_F ==
  slip_F : Inport
  Constant{1,3..8} (7 alike) : Constant  Value=0  OutDataTypeStr=uint8  SampleTime=-1
  slip_FABS : Abs
  slip_FCS : ArithShift  BitShiftNumber=-8
  slip_FConS : Constant  OutDataTypeStr=single
  slip_FCosR : Constant  Value=0  OutDataTypeStr=uint8
  slip_FROP : RelationalOperator  Operator=<  OutDataTypeStr=boolean
  slip_FRon : Rounding  Operator=round
  slip_FSW : Switch  Criteria=u2 ~= 0
  slip_F_1sat : Saturate  UpperLimit=255  LowerLimit=0
  slip_F_Convert : DataTypeConversion  OutDataTypeStr=uint8
  slip_F_Convert1 : DataTypeConversion  OutDataTypeStr=uint32
  slip_F_D : Product  Inputs=*/
  slip_F_F : Constant  OutDataTypeStr=single
  slip_F_L : simulink/Logic and Bit Operations/Bitwise Operator  logicop=AND  UseBitMask=on  BitMask=255  BitMaskRealWorld=Stored Integer
  slip_F_O : Constant  Value=0  OutDataTypeStr=single
  slip_F_S : ArithShift
  slip_F_sat : Saturate  UpperLimit=255  LowerLimit=0
  slip_F_st : Sum  Inputs=+-
  slip_Fsubcon : Sum  Inputs=+-
  output1 : Outport
  output2 : Outport  Port=2
  output3 : Outport  Port=3
  output4 : Outport  Port=4
  output5 : Outport  Port=5
  output6 : Outport  Port=6
  output7 : Outport  Port=7
  output8 : Outport  Port=8
  wires:
  Constant8/1 -> output8/1
  Constant7/1 -> output7/1
  Constant6/1 -> output6/1
  Constant5/1 -> output5/1
  Constant4/1 -> output4/1
  Constant3/1 -> output3/1
  Constant1/1 -> output1/1
  slip_F_Convert/1 -> output2/1
  slip_F_L/1 -> slip_F_Convert/1
  slip_F_Convert1/1 -> slip_F_L/1
  slip_F_1sat/1 -> slip_F_Convert1/1
  slip_F_S/1 -> slip_F_1sat/1
  slip_FSW/1 -> slip_F_S/1
  slip_FROP/1 -> slip_FSW/2
  slip_Fsubcon/1 -> slip_FSW/1
  slip_FABS/1 -> slip_Fsubcon/2
  slip_FCS/1 -> slip_Fsubcon/1
  slip_FConS/1 -> slip_FCS/1
  slip_FCosR/1 -> slip_FROP/2
  slip_FRon/1 -> slip_FSW/3, slip_FABS/1, slip_FROP/1
  slip_F_D/1 -> slip_FRon/1
  slip_F_F/1 -> slip_F_D/2
  slip_F_st/1 -> slip_F_D/1
  slip_F_O/1 -> slip_F_st/2
  slip_F_sat/1 -> slip_F_st/1
  slip_F/1 -> slip_F_sat/1

== system 21-E/ECU_can/ECU_dyn1/slip_R ==
  slip_R : Inport
  Constant{1..2,4..8} (7 alike) : Constant  Value=0  OutDataTypeStr=uint8  SampleTime=-1
  slip_RABS : Abs
  slip_RCS : ArithShift  BitShiftNumber=-8
  slip_RConS : Constant  OutDataTypeStr=single
  slip_RCosR : Constant  Value=0  OutDataTypeStr=uint8
  slip_RROP : RelationalOperator  Operator=<  OutDataTypeStr=boolean
  slip_RRon : Rounding  Operator=round
  slip_RSW : Switch  Criteria=u2 ~= 0
  slip_R_1sat : Saturate  UpperLimit=255  LowerLimit=0
  slip_R_Convert : DataTypeConversion  OutDataTypeStr=uint8
  slip_R_Convert1 : DataTypeConversion  OutDataTypeStr=uint32
  slip_R_D : Product  Inputs=*/
  slip_R_F : Constant  OutDataTypeStr=single
  slip_R_L : simulink/Logic and Bit Operations/Bitwise Operator  logicop=AND  UseBitMask=on  BitMask=255  BitMaskRealWorld=Stored Integer
  slip_R_O : Constant  Value=0  OutDataTypeStr=single
  slip_R_S : ArithShift
  slip_R_sat : Saturate  UpperLimit=255  LowerLimit=0
  slip_R_st : Sum  Inputs=+-
  slip_Rsubcon : Sum  Inputs=+-
  output1 : Outport
  output2 : Outport  Port=2
  output3 : Outport  Port=3
  output4 : Outport  Port=4
  output5 : Outport  Port=5
  output6 : Outport  Port=6
  output7 : Outport  Port=7
  output8 : Outport  Port=8
  wires:
  Constant8/1 -> output8/1
  Constant7/1 -> output7/1
  Constant6/1 -> output6/1
  Constant5/1 -> output5/1
  Constant4/1 -> output4/1
  Constant2/1 -> output2/1
  Constant1/1 -> output1/1
  slip_R_Convert/1 -> output3/1
  slip_R_L/1 -> slip_R_Convert/1
  slip_R_Convert1/1 -> slip_R_L/1
  slip_R_1sat/1 -> slip_R_Convert1/1
  slip_R_S/1 -> slip_R_1sat/1
  slip_RSW/1 -> slip_R_S/1
  slip_RROP/1 -> slip_RSW/2
  slip_Rsubcon/1 -> slip_RSW/1
  slip_RABS/1 -> slip_Rsubcon/2
  slip_RCS/1 -> slip_Rsubcon/1
  slip_RConS/1 -> slip_RCS/1
  slip_RCosR/1 -> slip_RROP/2
  slip_RRon/1 -> slip_RSW/3, slip_RABS/1, slip_RROP/1
  slip_R_D/1 -> slip_RRon/1
  slip_R_F/1 -> slip_R_D/2
  slip_R_st/1 -> slip_R_D/1
  slip_R_O/1 -> slip_R_st/2
  slip_R_sat/1 -> slip_R_st/1
  slip_R/1 -> slip_R_sat/1

== system 21-E/ECU_can/ECU_dyn1/speed ==
  speed : Inport
  Constant{2..8} (7 alike) : Constant  Value=0  OutDataTypeStr=uint8  SampleTime=-1
  speedRon : Rounding  Operator=round
  speed_1sat : Saturate  UpperLimit=255  LowerLimit=0
  speed_Convert : DataTypeConversion  OutDataTypeStr=uint8
  speed_Convert1 : DataTypeConversion  OutDataTypeStr=uint32
  speed_D : Product  Inputs=*/
  speed_F : Constant  OutDataTypeStr=single
  speed_L : simulink/Logic and Bit Operations/Bitwise Operator  logicop=AND  UseBitMask=on  BitMask=255  BitMaskRealWorld=Stored Integer
  speed_O : Constant  Value=0  OutDataTypeStr=single
  speed_S : ArithShift
  speed_sat : Saturate  UpperLimit=255  LowerLimit=0
  speed_st : Sum  Inputs=+-
  output1 : Outport
  output2 : Outport  Port=2
  output3 : Outport  Port=3
  output4 : Outport  Port=4
  output5 : Outport  Port=5
  output6 : Outport  Port=6
  output7 : Outport  Port=7
  output8 : Outport  Port=8
  wires:
  Constant8/1 -> output8/1
  Constant7/1 -> output7/1
  Constant6/1 -> output6/1
  Constant5/1 -> output5/1
  Constant4/1 -> output4/1
  Constant3/1 -> output3/1
  Constant2/1 -> output2/1
  speed_Convert/1 -> output1/1
  speed_L/1 -> speed_Convert/1
  speed_Convert1/1 -> speed_L/1
  speed_1sat/1 -> speed_Convert1/1
  speed_S/1 -> speed_1sat/1
  speedRon/1 -> speed_S/1
  speed_D/1 -> speedRon/1
  speed_F/1 -> speed_D/2
  speed_st/1 -> speed_D/1
  speed_O/1 -> speed_st/2
  speed_sat/1 -> speed_st/1
  speed/1 -> speed_sat/1

== system 21-E/ECU_can/ECU_sig1/acc_a ==
  acc_a : Inport
  Constant{1..4,6..8} (7 alike) : Constant  Value=0  OutDataTypeStr=uint8  SampleTime=-1
  acc_aRon : Rounding  Operator=round
  acc_a_1sat : Saturate  UpperLimit=255  LowerLimit=0
  acc_a_Convert : DataTypeConversion  OutDataTypeStr=uint8
  acc_a_Convert1 : DataTypeConversion  OutDataTypeStr=uint32
  acc_a_D : Product  Inputs=*/
  acc_a_F : Constant  OutDataTypeStr=single
  acc_a_L : simulink/Logic and Bit Operations/Bitwise Operator  logicop=AND  UseBitMask=on  BitMask=255  BitMaskRealWorld=Stored Integer
  acc_a_O : Constant  Value=0  OutDataTypeStr=single
  acc_a_S : ArithShift
  acc_a_sat : Saturate  UpperLimit=255  LowerLimit=0
  acc_a_st : Sum  Inputs=+-
  output1 : Outport
  output2 : Outport  Port=2
  output3 : Outport  Port=3
  output4 : Outport  Port=4
  output5 : Outport  Port=5
  output6 : Outport  Port=6
  output7 : Outport  Port=7
  output8 : Outport  Port=8
  wires:
  Constant8/1 -> output8/1
  Constant7/1 -> output7/1
  Constant6/1 -> output6/1
  Constant4/1 -> output4/1
  Constant3/1 -> output3/1
  Constant2/1 -> output2/1
  Constant1/1 -> output1/1
  acc_a_Convert/1 -> output5/1
  acc_a_L/1 -> acc_a_Convert/1
  acc_a_Convert1/1 -> acc_a_L/1
  acc_a_1sat/1 -> acc_a_Convert1/1
  acc_a_S/1 -> acc_a_1sat/1
  acc_aRon/1 -> acc_a_S/1
  acc_a_D/1 -> acc_aRon/1
  acc_a_F/1 -> acc_a_D/2
  acc_a_st/1 -> acc_a_D/1
  acc_a_O/1 -> acc_a_st/2
  acc_a_sat/1 -> acc_a_st/1
  acc_a/1 -> acc_a_sat/1

== system 21-E/ECU_can/ECU_sig1/acc_l ==
  acc_l : Inport
  Constant{1..3,5..8} (7 alike) : Constant  Value=0  OutDataTypeStr=uint8  SampleTime=-1
  acc_lRon : Rounding  Operator=round
  acc_l_1sat : Saturate  UpperLimit=255  LowerLimit=0
  acc_l_Convert : DataTypeConversion  OutDataTypeStr=uint8
  acc_l_Convert1 : DataTypeConversion  OutDataTypeStr=uint32
  acc_l_D : Product  Inputs=*/
  acc_l_F : Constant  OutDataTypeStr=single
  acc_l_L : simulink/Logic and Bit Operations/Bitwise Operator  logicop=AND  UseBitMask=on  BitMask=255  BitMaskRealWorld=Stored Integer
  acc_l_O : Constant  Value=0  OutDataTypeStr=single
  acc_l_S : ArithShift
  acc_l_sat : Saturate  UpperLimit=255  LowerLimit=0
  acc_l_st : Sum  Inputs=+-
  output1 : Outport
  output2 : Outport  Port=2
  output3 : Outport  Port=3
  output4 : Outport  Port=4
  output5 : Outport  Port=5
  output6 : Outport  Port=6
  output7 : Outport  Port=7
  output8 : Outport  Port=8
  wires:
  Constant8/1 -> output8/1
  Constant7/1 -> output7/1
  Constant6/1 -> output6/1
  Constant5/1 -> output5/1
  Constant3/1 -> output3/1
  Constant2/1 -> output2/1
  Constant1/1 -> output1/1
  acc_l_Convert/1 -> output4/1
  acc_l_L/1 -> acc_l_Convert/1
  acc_l_Convert1/1 -> acc_l_L/1
  acc_l_1sat/1 -> acc_l_Convert1/1
  acc_l_S/1 -> acc_l_1sat/1
  acc_lRon/1 -> acc_l_S/1
  acc_l_D/1 -> acc_lRon/1
  acc_l_F/1 -> acc_l_D/2
  acc_l_st/1 -> acc_l_D/1
  acc_l_O/1 -> acc_l_st/2
  acc_l_sat/1 -> acc_l_st/1
  acc_l/1 -> acc_l_sat/1

== system 21-E/ECU_can/ECU_sig1/angle ==
  angle : Inport
  Constant{2..8} (7 alike) : Constant  Value=0  OutDataTypeStr=uint8  SampleTime=-1
  angleABS : Abs
  angleCS : ArithShift  BitShiftNumber=-8
  angleConS : Constant  OutDataTypeStr=single
  angleCosR : Constant  Value=0  OutDataTypeStr=uint8
  angleROP : RelationalOperator  Operator=<  OutDataTypeStr=boolean
  angleRon : Rounding  Operator=round
  angleSW : Switch  Criteria=u2 ~= 0
  angle_1sat : Saturate  UpperLimit=255  LowerLimit=0
  angle_Convert : DataTypeConversion  OutDataTypeStr=uint8
  angle_Convert1 : DataTypeConversion  OutDataTypeStr=uint32
  angle_D : Product  Inputs=*/
  angle_F : Constant  OutDataTypeStr=single
  angle_L : simulink/Logic and Bit Operations/Bitwise Operator  logicop=AND  UseBitMask=on  BitMask=255  BitMaskRealWorld=Stored Integer
  angle_O : Constant  Value=0  OutDataTypeStr=single
  angle_S : ArithShift
  angle_sat : Saturate  UpperLimit=255  LowerLimit=0
  angle_st : Sum  Inputs=+-
  anglesubcon : Sum  Inputs=+-
  output1 : Outport
  output2 : Outport  Port=2
  output3 : Outport  Port=3
  output4 : Outport  Port=4
  output5 : Outport  Port=5
  output6 : Outport  Port=6
  output7 : Outport  Port=7
  output8 : Outport  Port=8
  wires:
  Constant8/1 -> output8/1
  Constant7/1 -> output7/1
  Constant6/1 -> output6/1
  Constant5/1 -> output5/1
  Constant4/1 -> output4/1
  Constant3/1 -> output3/1
  Constant2/1 -> output2/1
  angle_Convert/1 -> output1/1
  angle_L/1 -> angle_Convert/1
  angle_Convert1/1 -> angle_L/1
  angle_1sat/1 -> angle_Convert1/1
  angle_S/1 -> angle_1sat/1
  angleSW/1 -> angle_S/1
  angleROP/1 -> angleSW/2
  anglesubcon/1 -> angleSW/1
  angleABS/1 -> anglesubcon/2
  angleCS/1 -> anglesubcon/1
  angleConS/1 -> angleCS/1
  angleCosR/1 -> angleROP/2
  angleRon/1 -> angleSW/3, angleABS/1, angleROP/1
  angle_D/1 -> angleRon/1
  angle_F/1 -> angle_D/2
  angle_st/1 -> angle_D/1
  angle_O/1 -> angle_st/2
  angle_sat/1 -> angle_st/1
  angle/1 -> angle_sat/1

== system 21-E/ECU_can/ECU_sig1/bre_l ==
  bre_l : Inport
  Constant{1..5,7..8} (7 alike) : Constant  Value=0  OutDataTypeStr=uint8  SampleTime=-1
  bre_lRon : Rounding  Operator=round
  bre_l_1sat : Saturate  UpperLimit=255  LowerLimit=0
  bre_l_Convert : DataTypeConversion  OutDataTypeStr=uint8
  bre_l_Convert1 : DataTypeConversion  OutDataTypeStr=uint32
  bre_l_D : Product  Inputs=*/
  bre_l_F : Constant  OutDataTypeStr=single
  bre_l_L : simulink/Logic and Bit Operations/Bitwise Operator  logicop=AND  UseBitMask=on  BitMask=255  BitMaskRealWorld=Stored Integer
  bre_l_O : Constant  Value=0  OutDataTypeStr=single
  bre_l_S : ArithShift
  bre_l_sat : Saturate  UpperLimit=255  LowerLimit=0
  bre_l_st : Sum  Inputs=+-
  output1 : Outport
  output2 : Outport  Port=2
  output3 : Outport  Port=3
  output4 : Outport  Port=4
  output5 : Outport  Port=5
  output6 : Outport  Port=6
  output7 : Outport  Port=7
  output8 : Outport  Port=8
  wires:
  Constant8/1 -> output8/1
  Constant7/1 -> output7/1
  Constant5/1 -> output5/1
  Constant4/1 -> output4/1
  Constant3/1 -> output3/1
  Constant2/1 -> output2/1
  Constant1/1 -> output1/1
  bre_l_Convert/1 -> output6/1
  bre_l_L/1 -> bre_l_Convert/1
  bre_l_Convert1/1 -> bre_l_L/1
  bre_l_1sat/1 -> bre_l_Convert1/1
  bre_l_S/1 -> bre_l_1sat/1
  bre_lRon/1 -> bre_l_S/1
  bre_l_D/1 -> bre_lRon/1
  bre_l_F/1 -> bre_l_D/2
  bre_l_st/1 -> bre_l_D/1
  bre_l_O/1 -> bre_l_st/2
  bre_l_sat/1 -> bre_l_st/1
  bre_l/1 -> bre_l_sat/1

== system 21-E/ECU_can/ECU_sig1/bre_o_1 ==
  bre_o_1 : Inport
  Constant{1..6,8} (7 alike) : Constant  Value=0  OutDataTypeStr=uint8  SampleTime=-1
  bre_o_1Ron : Rounding  Operator=round
  bre_o_1_1sat : Saturate  UpperLimit=255  LowerLimit=0
  bre_o_1_Convert : DataTypeConversion  OutDataTypeStr=uint8
  bre_o_1_Convert1 : DataTypeConversion  OutDataTypeStr=uint32
  bre_o_1_D : Product  Inputs=*/
  bre_o_1_F : Constant  OutDataTypeStr=single
  bre_o_1_L : simulink/Logic and Bit Operations/Bitwise Operator  logicop=AND  UseBitMask=on  BitMask=255  BitMaskRealWorld=Stored Integer
  bre_o_1_O : Constant  Value=0  OutDataTypeStr=single
  bre_o_1_S : ArithShift
  bre_o_1_sat : Saturate  UpperLimit=255  LowerLimit=0
  bre_o_1_st : Sum  Inputs=+-
  output1 : Outport
  output2 : Outport  Port=2
  output3 : Outport  Port=3
  output4 : Outport  Port=4
  output5 : Outport  Port=5
  output6 : Outport  Port=6
  output7 : Outport  Port=7
  output8 : Outport  Port=8
  wires:
  Constant8/1 -> output8/1
  Constant6/1 -> output6/1
  Constant5/1 -> output5/1
  Constant4/1 -> output4/1
  Constant3/1 -> output3/1
  Constant2/1 -> output2/1
  Constant1/1 -> output1/1
  bre_o_1_Convert/1 -> output7/1
  bre_o_1_L/1 -> bre_o_1_Convert/1
  bre_o_1_Convert1/1 -> bre_o_1_L/1
  bre_o_1_1sat/1 -> bre_o_1_Convert1/1
  bre_o_1_S/1 -> bre_o_1_1sat/1
  bre_o_1Ron/1 -> bre_o_1_S/1
  bre_o_1_D/1 -> bre_o_1Ron/1
  bre_o_1_F/1 -> bre_o_1_D/2
  bre_o_1_st/1 -> bre_o_1_D/1
  bre_o_1_O/1 -> bre_o_1_st/2
  bre_o_1_sat/1 -> bre_o_1_st/1
  bre_o_1/1 -> bre_o_1_sat/1

== system 21-E/ECU_can/ECU_sig1/bre_o_2 ==
  bre_o_2 : Inport
  Constant{1..7} (7 alike) : Constant  Value=0  OutDataTypeStr=uint8  SampleTime=-1
  bre_o_2Ron : Rounding  Operator=round
  bre_o_2_1sat : Saturate  UpperLimit=255  LowerLimit=0
  bre_o_2_Convert : DataTypeConversion  OutDataTypeStr=uint8
  bre_o_2_Convert1 : DataTypeConversion  OutDataTypeStr=uint32
  bre_o_2_D : Product  Inputs=*/
  bre_o_2_F : Constant  OutDataTypeStr=single
  bre_o_2_L : simulink/Logic and Bit Operations/Bitwise Operator  logicop=AND  UseBitMask=on  BitMask=255  BitMaskRealWorld=Stored Integer
  bre_o_2_O : Constant  Value=0  OutDataTypeStr=single
  bre_o_2_S : ArithShift
  bre_o_2_sat : Saturate  UpperLimit=255  LowerLimit=0
  bre_o_2_st : Sum  Inputs=+-
  output1 : Outport
  output2 : Outport  Port=2
  output3 : Outport  Port=3
  output4 : Outport  Port=4
  output5 : Outport  Port=5
  output6 : Outport  Port=6
  output7 : Outport  Port=7
  output8 : Outport  Port=8
  wires:
  Constant7/1 -> output7/1
  Constant6/1 -> output6/1
  Constant5/1 -> output5/1
  Constant4/1 -> output4/1
  Constant3/1 -> output3/1
  Constant2/1 -> output2/1
  Constant1/1 -> output1/1
  bre_o_2_Convert/1 -> output8/1
  bre_o_2_L/1 -> bre_o_2_Convert/1
  bre_o_2_Convert1/1 -> bre_o_2_L/1
  bre_o_2_1sat/1 -> bre_o_2_Convert1/1
  bre_o_2_S/1 -> bre_o_2_1sat/1
  bre_o_2Ron/1 -> bre_o_2_S/1
  bre_o_2_D/1 -> bre_o_2Ron/1
  bre_o_2_F/1 -> bre_o_2_D/2
  bre_o_2_st/1 -> bre_o_2_D/1
  bre_o_2_O/1 -> bre_o_2_st/2
  bre_o_2_sat/1 -> bre_o_2_st/1
  bre_o_2/1 -> bre_o_2_sat/1

== system 21-E/ECU_can/ECU_sig1/yaw_i ==
  yaw_i : Inport
  Constant{1,3..8} (7 alike) : Constant  Value=0  OutDataTypeStr=uint8  SampleTime=-1
  yaw_iABS : Abs
  yaw_iCS : ArithShift  BitShiftNumber=-8
  yaw_iConS : Constant  OutDataTypeStr=single
  yaw_iCosR : Constant  Value=0  OutDataTypeStr=uint8
  yaw_iROP : RelationalOperator  Operator=<  OutDataTypeStr=boolean
  yaw_iRon : Rounding  Operator=round
  yaw_iSW : Switch  Criteria=u2 ~= 0
  yaw_i_1sat : Saturate  UpperLimit=255  LowerLimit=0
  yaw_i_Convert : DataTypeConversion  OutDataTypeStr=uint8
  yaw_i_Convert1 : DataTypeConversion  OutDataTypeStr=uint32
  yaw_i_D : Product  Inputs=*/
  yaw_i_F : Constant  OutDataTypeStr=single
  yaw_i_L : simulink/Logic and Bit Operations/Bitwise Operator  logicop=AND  UseBitMask=on  BitMask=255  BitMaskRealWorld=Stored Integer
  yaw_i_O : Constant  Value=0  OutDataTypeStr=single
  yaw_i_S : ArithShift
  yaw_i_sat : Saturate  UpperLimit=255  LowerLimit=0
  yaw_i_st : Sum  Inputs=+-
  yaw_isubcon : Sum  Inputs=+-
  output1 : Outport
  output2 : Outport  Port=2
  output3 : Outport  Port=3
  output4 : Outport  Port=4
  output5 : Outport  Port=5
  output6 : Outport  Port=6
  output7 : Outport  Port=7
  output8 : Outport  Port=8
  wires:
  Constant8/1 -> output8/1
  Constant7/1 -> output7/1
  Constant6/1 -> output6/1
  Constant5/1 -> output5/1
  Constant4/1 -> output4/1
  Constant3/1 -> output3/1
  Constant1/1 -> output1/1
  yaw_i_Convert/1 -> output2/1
  yaw_i_L/1 -> yaw_i_Convert/1
  yaw_i_Convert1/1 -> yaw_i_L/1
  yaw_i_1sat/1 -> yaw_i_Convert1/1
  yaw_i_S/1 -> yaw_i_1sat/1
  yaw_iSW/1 -> yaw_i_S/1
  yaw_iROP/1 -> yaw_iSW/2
  yaw_isubcon/1 -> yaw_iSW/1
  yaw_iABS/1 -> yaw_isubcon/2
  yaw_iCS/1 -> yaw_isubcon/1
  yaw_iConS/1 -> yaw_iCS/1
  yaw_iCosR/1 -> yaw_iROP/2
  yaw_iRon/1 -> yaw_iSW/3, yaw_iABS/1, yaw_iROP/1
  yaw_i_D/1 -> yaw_iRon/1
  yaw_i_F/1 -> yaw_i_D/2
  yaw_i_st/1 -> yaw_i_D/1
  yaw_i_O/1 -> yaw_i_st/2
  yaw_i_sat/1 -> yaw_i_st/1
  yaw_i/1 -> yaw_i_sat/1
